simulink model "ElasticModel"  (R2018a)
settings: Solver=ode45  StartTime=0.0  StopTime=1  MaxStep=1e-4  MinStep=1e-6  RelTol=1e-4  AbsTol=1e-7
settings Model: Creator=thoma_000  LastModifiedBy=thoma_000
settings SolverCC: ZeroCrossAlgorithm=Adaptive
settings DebuggingCC: MaxConsecutiveZCsMsg=none

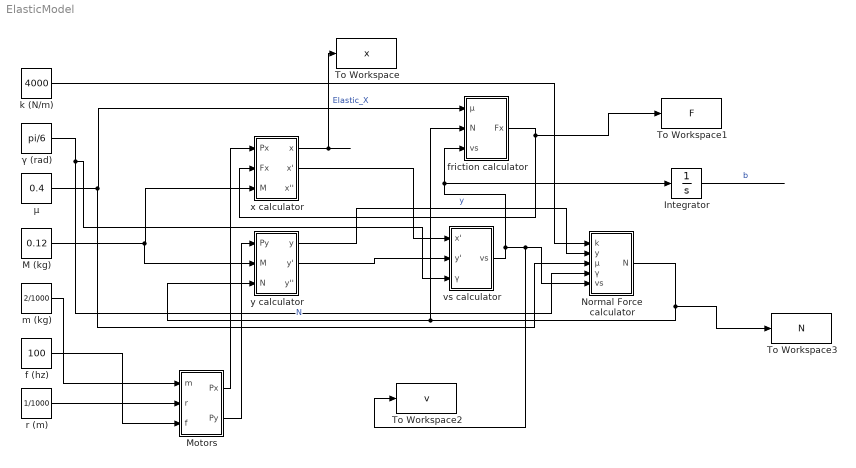
== system ElasticModel ==
  Integrator : Integrator
  M (kg) : Constant  Value=0.12
  Motors : Subsystem
  Normal Force calculator : Subsystem
  To Workspace : ToWorkspace  VariableName=x  SaveFormat=Timeseries  SampleTime=-1
      settings: Decimation=10
  To Workspace1 : ToWorkspace  VariableName=F  SaveFormat=Timeseries  SampleTime=-1
      settings: Decimation=10
  To Workspace2 : ToWorkspace  VariableName=v  SaveFormat=Timeseries  SampleTime=-1
      settings: Decimation=10
  To Workspace3 : ToWorkspace  VariableName=N  SaveFormat=Timeseries  SampleTime=-1
      settings: Decimation=10
  f (hz) : Constant  Value=100
  friction calculator : Subsystem
  k (N/m) : Constant  Value=4000
  m (kg) : Constant  Value=2/1000
  r (m) : Constant  Value=1/1000
  vs calculator : Subsystem
  x calculator : Subsystem
  y calculator : Subsystem
  γ (rad) : Constant  Value=pi/6
  μ : Constant  Value=0.4
  wires:
  y calculator/2(y') -> vs calculator/2(y')
  x calculator/2(x') -> vs calculator/1(x')
  friction calculator/1(Fx) -> To Workspace1/1, x calculator/2(Fx)
  M (kg)/1 -> y calculator/2(M), x calculator/3(M)
  vs calculator/1(vs) -> To Workspace2/1, Normal Force calculator/5(vs), Integrator/1, friction calculator/3(vs)
  μ/1 -> Normal Force calculator/3(μ), friction calculator/1(μ)
  γ (rad)/1 -> vs calculator/3(γ), Normal Force calculator/4(γ)
  y calculator/1(y) -> Normal Force calculator/2(y)  "y"
  k (N/m)/1 -> Normal Force calculator/1(k)
  Motors/1(Px) -> x calculator/1(Px)
  Motors/2(Py) -> y calculator/1(Py)
  m (kg)/1 -> Motors/1(m)
  r (m)/1 -> Motors/2(r)
  f (hz)/1 -> Motors/3(f)
  Normal Force calculator/1(N) -> To Workspace3/1, y calculator/3(N), friction calculator/2(N)  "N"
  x calculator/1(x) -> To Workspace/1  "Elastic_X"
  Integrator/1 -> ?  "b"

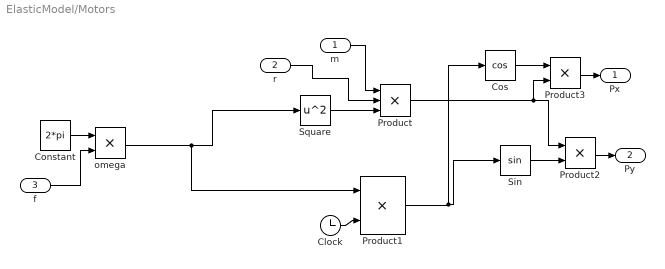
== system ElasticModel/Motors ==
  m : Inport
  r : Inport  Port=2
  f : Inport  Port=3
  Clock : Clock
  Constant : Constant  Value=2*pi
  Cos : Trigonometry  Operator=cos
  Product : Product  Inputs=***
  Product1 : Product
  Product2 : Product
  Product3 : Product
  Sin : Trigonometry
  Square : Math  Operator=square  SaturateOnIntegerOverflow=on
  omega : Product
  Px : Outport
  Py : Outport  Port=2
  wires:
  Cos/1 -> Product3/1
  Product/1 -> Product2/1, Product3/2
  Product1/1 -> Sin/1, Cos/1
  Square/1 -> Product/3
  Clock/1 -> Product1/2
  Sin/1 -> Product2/2
  Product3/1 -> Px/1
  Product2/1 -> Py/1
  r/1 -> Product/2
  m/1 -> Product/1
  Constant/1 -> omega/1
  f/1 -> omega/2
  omega/1 -> Product1/1, Square/1

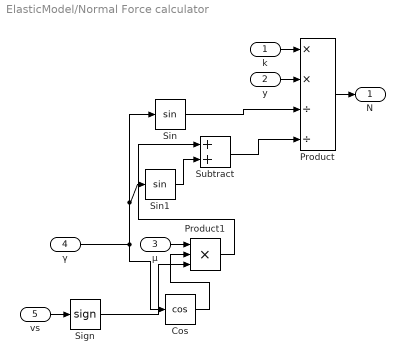
== system ElasticModel/Normal Force calculator ==
  k : Inport
  y : Inport  Port=2
  μ : Inport  Port=3
  γ : Inport  Port=4
  vs : Inport  Port=5
  Cos : Trigonometry  Operator=cos
  Product : Product  Inputs=**//
  Product1 : Product  Inputs=***
  Sign : Signum
  Sin : Trigonometry
  Sin1 : Trigonometry
  Subtract : Sum
  N : Outport
  wires:
  Product1/1 -> Subtract/1
  Sin1/1 -> Subtract/2
  Sign/1 -> Product1/3
  μ/1 -> Product1/1
  γ/1 -> Cos/1, Sin1/1, Sin/1
  Subtract/1 -> Product/4
  Sin/1 -> Product/3
  Cos/1 -> Product1/2
  Product/1 -> N/1
  y/1 -> Product/2
  vs/1 -> Sign/1
  k/1 -> Product/1

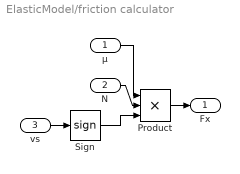
== system ElasticModel/friction calculator ==
  μ : Inport
  N : Inport  Port=2
  vs : Inport  Port=3
  Product : Product  Inputs=***
  Sign : Signum
  Fx : Outport
  wires:
  Sign/1 -> Product/3
  μ/1 -> Product/1
  Product/1 -> Fx/1
  N/1 -> Product/2
  vs/1 -> Sign/1

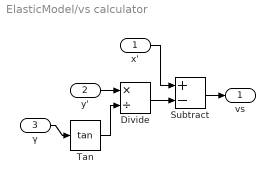
== system ElasticModel/vs calculator ==
  x' : Inport
  y' : Inport  Port=2
  γ : Inport  Port=3
  Divide : Product  Inputs=*/
  Subtract : Sum  Inputs=+-
  Tan : Trigonometry  Operator=tan
  vs : Outport
  wires:
  y'/1 -> Divide/1
  Subtract/1 -> vs/1
  Divide/1 -> Subtract/2
  x'/1 -> Subtract/1
  γ/1 -> Tan/1
  Tan/1 -> Divide/2

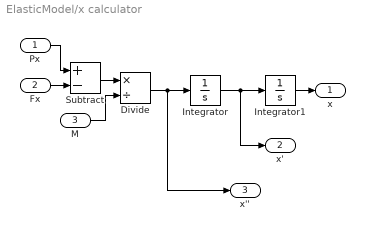
== system ElasticModel/x calculator ==
  Px : Inport
  Fx : Inport  Port=2
  M : Inport  Port=3
  Divide : Product  Inputs=*/
  Integrator : Integrator
  Integrator1 : Integrator
  Subtract : Sum  Inputs=+-
  x : Outport
  x' : Outport  Port=2
  x'' : Outport  Port=3
  wires:
  Px/1 -> Subtract/1
  Divide/1 -> x''/1, Integrator/1
  Integrator/1 -> x'/1, Integrator1/1
  Fx/1 -> Subtract/2
  M/1 -> Divide/2
  Integrator1/1 -> x/1
  Subtract/1 -> Divide/1

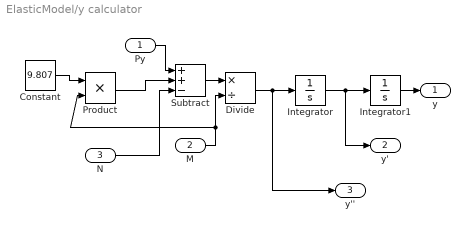
== system ElasticModel/y calculator ==
  Py : Inport
  M : Inport  Port=2
  N : Inport  Port=3
  Constant : Constant  Value=9.807
  Divide : Product  Inputs=*/
  Integrator : Integrator
  Integrator1 : Integrator
  Product : Product
  Subtract : Sum  Inputs=++-
  y : Outport
  y' : Outport  Port=2
  y'' : Outport  Port=3
  wires:
  Py/1 -> Subtract/1
  Divide/1 -> y''/1, Integrator/1
  Integrator/1 -> y'/1, Integrator1/1
  Product/1 -> Subtract/2
  M/1 -> Product/2, Divide/2
  Integrator1/1 -> y/1
  Subtract/1 -> Divide/1
  Constant/1 -> Product/1
  N/1 -> Subtract/3
